simulink model "Static_Deflection_State_Space"  (R2016a)
settings: Solver=ode23t  StartTime=0.0  StopTime=100  RelTol=1e-3
InitFcn:
  | %if ~exist('linsys_beam_fixfree','var') ||~exist('linsys_beam_rotfree','var')
  |    load SS_Damping_1e7.mat
  |    disp('State Space Models does not exist in workspace, loading presaved SS models')
  | %end
StopFcn:
  | disp(['Static Deflection is ' num2str(SS_Def.signals.values(end)) ' m'])
undefined symbols (not defined in the file): beam_wall, beam_width, density, element_length, gravity, num_elem
libraries: cstblocks x1
Description:
  | Copyright 2014-2016 The MathWorks, Inc.
settings Model: Creator=psanghvi  LastModifiedBy=smiller
settings DataIOCC: LimitDataPoints=on  SaveFormat=Array
settings DebuggingCC: UnderspecifiedInitializationDetection=Classic  MergeDetectMultiDrivingBlocksExec=none  SolverPrmCheckMsg=warning  AllowSymbolicDim=off
settings HardwareCC: ProdBitPerPointer=32  ProdLargestAtomicFloat=None  ProdIntDivRoundTo=Undefined  ProdEndianess=Unspecified  ProdWordSize=32  ProdHWDeviceType=32-bit Generic
settings ModelReferenceCC: PropagateSignalLabelsOutOfModel=off
settings ConfigComp: CovModelRefEnable=Off  CovSFcnEnable=off

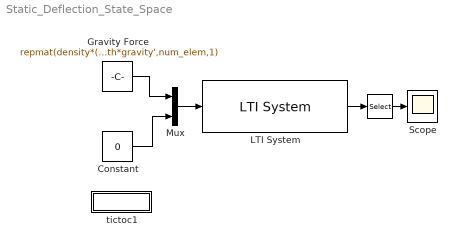
== system Static_Deflection_State_Space ==
  "  " : Selector  InputPortWidth=num_elem+1  IndexOptions=Index vector (dialog)  Indices=num_elem+1  OutputSizes=1
  Constant : Constant  Value=0
  Gravity Force : Constant  Value=repmat(density*(beam_width^2- (beam_width-beam_wall*2)^2)*element_length*gravity',num_elem,1)
  LTI System : cstblocks/LTI System  sys=linsys_beam_fixfree  IC=[]
  Mux : Mux  Inputs=2
  Scope : Scope
  tictoc1 : Subsystem
      settings: OpenFcn=open('Flexible_Beam_Demo_Script.html')
      mask Display: disp('Script')
  wires:
  Constant/1 -> Mux/2
  Gravity Force/1 -> Mux/1
  Mux/1 -> LTI System/1
  LTI System/1 -> "  "/1
  "  "/1 -> Scope/1

== system Static_Deflection_State_Space/tictoc1 ==
